simulink model "signal_tranmission"  (R2024b)
settings: Solver=ode45  StartTime=0.0  StopTime=10  FixedStep=0.000125  RelTol=1e-3
libraries: dspfdesign x500, commchan3 x1
(part 1 of 7)
settings Model: Creator=hp  LastModifiedBy=BHISMODEV

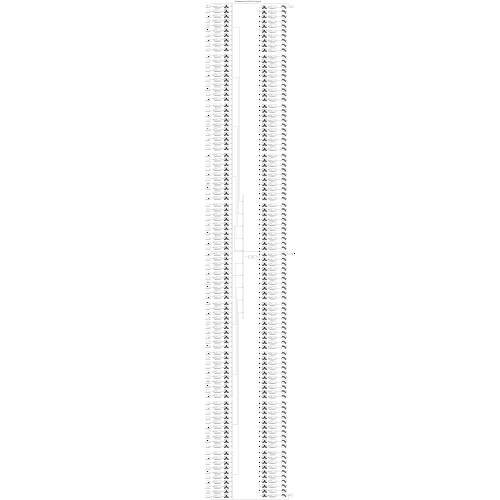
[thumbnail: Simulink's stored preview of the top-level diagram]
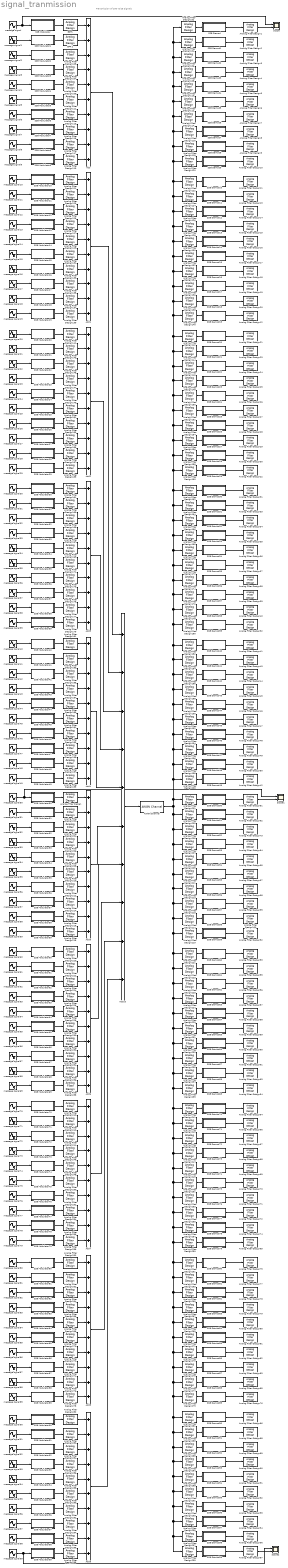
== system signal_tranmission ==
  note: Transmission of 100 Voice Signals
  AWGN Channel : commchan3/AWGN Channel  LegacyMode=off  NoiseMethod="Signal to noise ratio  (SNR)"  noiseMode="Signal to noise ratio  (SNR)"  EbNo=10  EsNo=10  SNR=80  BitsPerSymbol=1  SignalPower=1  SamplesPerSymbol=1  SymbolPeriod=1  VarianceSource=Parameter  Variance=1  RandomStream=Global stream  Seed=67  SimulateUsing=Interpreted execution
  Add{,1..10} (11 alike) : Sum  Inputs=10
  Analog Filter Design : dspfdesign/Analog Filter Design  method=Butterworth  filttype=Bandpass  N=4  Wlo=298*2*pi  Whi=302*2*pi  Rp=2  Rs=40
  Analog Filter Design{1..100} (100 alike) : dspfdesign/Analog Filter Design  method=Butterworth  filttype=Lowpass  N=4  Wlo=5*2*pi  Whi=102*2*pi  Rp=2  Rs=40
  Analog Filter Design102 : dspfdesign/Analog Filter Design  method=Butterworth  filttype=Bandpass  N=4  Wlo=98*2*pi  Whi=102*2*pi  Rp=2  Rs=40
  Analog Filter Design104 : dspfdesign/Analog Filter Design  method=Butterworth  filttype=Bandpass  N=4  Wlo=102*2*pi  Whi=106*2*pi  Rp=2  Rs=40
  Analog Filter Design105 : dspfdesign/Analog Filter Design  method=Butterworth  filttype=Bandpass  N=4  Wlo=106*2*pi  Whi=110*2*pi  Rp=2  Rs=40
  Analog Filter Design106 : dspfdesign/Analog Filter Design  method=Butterworth  filttype=Bandpass  N=4  Wlo=106*2*pi  Whi=110*2*pi  Rp=2  Rs=40
  Analog Filter Design107 : dspfdesign/Analog Filter Design  method=Butterworth  filttype=Bandpass  N=4  Wlo=110*2*pi  Whi=114*2*pi  Rp=2  Rs=40
  Analog Filter Design108 : dspfdesign/Analog Filter Design  method=Butterworth  filttype=Bandpass  N=4  Wlo=110*2*pi  Whi=114*2*pi  Rp=2  Rs=40
  Analog Filter Design109 : dspfdesign/Analog Filter Design  method=Butterworth  filttype=Bandpass  N=4  Wlo=114*2*pi  Whi=118*2*pi  Rp=2  Rs=40
  Analog Filter Design110 : dspfdesign/Analog Filter Design  method=Butterworth  filttype=Bandpass  N=4  Wlo=114*2*pi  Whi=118*2*pi  Rp=2  Rs=40
  Analog Filter Design111 : dspfdesign/Analog Filter Design  method=Butterworth  filttype=Bandpass  N=4  Wlo=118*2*pi  Whi=122*2*pi  Rp=2  Rs=40
  Analog Filter Design112 : dspfdesign/Analog Filter Design  method=Butterworth  filttype=Bandpass  N=4  Wlo=118*2*pi  Whi=122*2*pi  Rp=2  Rs=40
  Analog Filter Design113 : dspfdesign/Analog Filter Design  method=Butterworth  filttype=Bandpass  N=4  Wlo=122*2*pi  Whi=126*2*pi  Rp=2  Rs=40
  Analog Filter Design114 : dspfdesign/Analog Filter Design  method=Butterworth  filttype=Bandpass  N=4  Wlo=122*2*pi  Whi=126*2*pi  Rp=2  Rs=40
  Analog Filter Design115 : dspfdesign/Analog Filter Design  method=Butterworth  filttype=Bandpass  N=4  Wlo=126*2*pi  Whi=130*2*pi  Rp=2  Rs=40
  Analog Filter Design116 : dspfdesign/Analog Filter Design  method=Butterworth  filttype=Bandpass  N=4  Wlo=126*2*pi  Whi=130*2*pi  Rp=2  Rs=40
  Analog Filter Design117 : dspfdesign/Analog Filter Design  method=Butterworth  filttype=Bandpass  N=4  Wlo=130*2*pi  Whi=134*2*pi  Rp=2  Rs=40
  Analog Filter Design118 : dspfdesign/Analog Filter Design  method=Butterworth  filttype=Bandpass  N=4  Wlo=130*2*pi  Whi=134*2*pi  Rp=2  Rs=40
  Analog Filter Design119 : dspfdesign/Analog Filter Design  method=Butterworth  filttype=Bandpass  N=4  Wlo=134*2*pi  Whi=138*2*pi  Rp=2  Rs=40
  Analog Filter Design120 : dspfdesign/Analog Filter Design  method=Butterworth  filttype=Bandpass  N=4  Wlo=134*2*pi  Whi=138*2*pi  Rp=2  Rs=40
  Analog Filter Design121 : dspfdesign/Analog Filter Design  method=Butterworth  filttype=Bandpass  N=4  Wlo=138*2*pi  Whi=142*2*pi  Rp=2  Rs=40
  Analog Filter Design122 : dspfdesign/Analog Filter Design  method=Butterworth  filttype=Bandpass  N=4  Wlo=138*2*pi  Whi=142*2*pi  Rp=2  Rs=40
  Analog Filter Design123 : dspfdesign/Analog Filter Design  method=Butterworth  filttype=Bandpass  N=4  Wlo=142*2*pi  Whi=146*2*pi  Rp=2  Rs=40
  Analog Filter Design124 : dspfdesign/Analog Filter Design  method=Butterworth  filttype=Bandpass  N=4  Wlo=142*2*pi  Whi=146*2*pi  Rp=2  Rs=40
  Analog Filter Design125 : dspfdesign/Analog Filter Design  method=Butterworth  filttype=Bandpass  N=4  Wlo=146*2*pi  Whi=150*2*pi  Rp=2  Rs=40
  Analog Filter Design126 : dspfdesign/Analog Filter Design  method=Butterworth  filttype=Bandpass  N=4  Wlo=146*2*pi  Whi=150*2*pi  Rp=2  Rs=40
  Analog Filter Design127 : dspfdesign/Analog Filter Design  method=Butterworth  filttype=Bandpass  N=4  Wlo=150*2*pi  Whi=154*2*pi  Rp=2  Rs=40
  Analog Filter Design128 : dspfdesign/Analog Filter Design  method=Butterworth  filttype=Bandpass  N=4  Wlo=150*2*pi  Whi=154*2*pi  Rp=2  Rs=40
  Analog Filter Design129 : dspfdesign/Analog Filter Design  method=Butterworth  filttype=Bandpass  N=4  Wlo=154*2*pi  Whi=158*2*pi  Rp=2  Rs=40
  Analog Filter Design130 : dspfdesign/Analog Filter Design  method=Butterworth  filttype=Bandpass  N=4  Wlo=154*2*pi  Whi=158*2*pi  Rp=2  Rs=40
  Analog Filter Design131 : dspfdesign/Analog Filter Design  method=Butterworth  filttype=Bandpass  N=4  Wlo=158*2*pi  Whi=162*2*pi  Rp=2  Rs=40
  Analog Filter Design132 : dspfdesign/Analog Filter Design  method=Butterworth  filttype=Bandpass  N=4  Wlo=158*2*pi  Whi=162*2*pi  Rp=2  Rs=40
  Analog Filter Design133 : dspfdesign/Analog Filter Design  method=Butterworth  filttype=Bandpass  N=4  Wlo=162*2*pi  Whi=166*2*pi  Rp=2  Rs=40
  Analog Filter Design134 : dspfdesign/Analog Filter Design  method=Butterworth  filttype=Bandpass  N=4  Wlo=162*2*pi  Whi=166*2*pi  Rp=2  Rs=40
  Analog Filter Design135 : dspfdesign/Analog Filter Design  method=Butterworth  filttype=Bandpass  N=4  Wlo=166*2*pi  Whi=170*2*pi  Rp=2  Rs=40
  Analog Filter Design136 : dspfdesign/Analog Filter Design  method=Butterworth  filttype=Bandpass  N=4  Wlo=166*2*pi  Whi=170*2*pi  Rp=2  Rs=40
  Analog Filter Design137 : dspfdesign/Analog Filter Design  method=Butterworth  filttype=Bandpass  N=4  Wlo=170*2*pi  Whi=174*2*pi  Rp=2  Rs=40
  Analog Filter Design138 : dspfdesign/Analog Filter Design  method=Butterworth  filttype=Bandpass  N=4  Wlo=170*2*pi  Whi=174*2*pi  Rp=2  Rs=40
  Analog Filter Design139 : dspfdesign/Analog Filter Design  method=Butterworth  filttype=Bandpass  N=4  Wlo=174*2*pi  Whi=178*2*pi  Rp=2  Rs=40
  Analog Filter Design140 : dspfdesign/Analog Filter Design  method=Butterworth  filttype=Bandpass  N=4  Wlo=174*2*pi  Whi=178*2*pi  Rp=2  Rs=40
  Analog Filter Design141 : dspfdesign/Analog Filter Design  method=Butterworth  filttype=Bandpass  N=4  Wlo=178*2*pi  Whi=182*2*pi  Rp=2  Rs=40
  Analog Filter Design142 : dspfdesign/Analog Filter Design  method=Butterworth  filttype=Bandpass  N=4  Wlo=178*2*pi  Whi=182*2*pi  Rp=2  Rs=40
  Analog Filter Design143 : dspfdesign/Analog Filter Design  method=Butterworth  filttype=Bandpass  N=4  Wlo=182*2*pi  Whi=186*2*pi  Rp=2  Rs=40
  Analog Filter Design144 : dspfdesign/Analog Filter Design  method=Butterworth  filttype=Bandpass  N=4  Wlo=182*2*pi  Whi=186*2*pi  Rp=2  Rs=40
  Analog Filter Design145 : dspfdesign/Analog Filter Design  method=Butterworth  filttype=Bandpass  N=4  Wlo=186*2*pi  Whi=190*2*pi  Rp=2  Rs=40
  Analog Filter Design146 : dspfdesign/Analog Filter Design  method=Butterworth  filttype=Bandpass  N=4  Wlo=186*2*pi  Whi=190*2*pi  Rp=2  Rs=40
  Analog Filter Design147 : dspfdesign/Analog Filter Design  method=Butterworth  filttype=Bandpass  N=4  Wlo=190*2*pi  Whi=194*2*pi  Rp=2  Rs=40
  Analog Filter Design148 : dspfdesign/Analog Filter Design  method=Butterworth  filttype=Bandpass  N=4  Wlo=190*2*pi  Whi=194*2*pi  Rp=2  Rs=40
  Analog Filter Design149 : dspfdesign/Analog Filter Design  method=Butterworth  filttype=Bandpass  N=4  Wlo=194*2*pi  Whi=198*2*pi  Rp=2  Rs=40
  Analog Filter Design150 : dspfdesign/Analog Filter Design  method=Butterworth  filttype=Bandpass  N=4  Wlo=194*2*pi  Whi=198*2*pi  Rp=2  Rs=40
  Analog Filter Design151 : dspfdesign/Analog Filter Design  method=Butterworth  filttype=Bandpass  N=4  Wlo=198*2*pi  Whi=202*2*pi  Rp=2  Rs=40
  Analog Filter Design152 : dspfdesign/Analog Filter Design  method=Butterworth  filttype=Bandpass  N=4  Wlo=198*2*pi  Whi=202*2*pi  Rp=2  Rs=40
  Analog Filter Design153 : dspfdesign/Analog Filter Design  method=Butterworth  filttype=Bandpass  N=4  Wlo=202*2*pi  Whi=206*2*pi  Rp=2  Rs=40
  Analog Filter Design154 : dspfdesign/Analog Filter Design  method=Butterworth  filttype=Bandpass  N=4  Wlo=202*2*pi  Whi=206*2*pi  Rp=2  Rs=40
  Analog Filter Design155 : dspfdesign/Analog Filter Design  method=Butterworth  filttype=Bandpass  N=4  Wlo=206*2*pi  Whi=210*2*pi  Rp=2  Rs=40
  Analog Filter Design156 : dspfdesign/Analog Filter Design  method=Butterworth  filttype=Bandpass  N=4  Wlo=206*2*pi  Whi=210*2*pi  Rp=2  Rs=40
  Analog Filter Design157 : dspfdesign/Analog Filter Design  method=Butterworth  filttype=Bandpass  N=4  Wlo=210*2*pi  Whi=214*2*pi  Rp=2  Rs=40
  Analog Filter Design158 : dspfdesign/Analog Filter Design  method=Butterworth  filttype=Bandpass  N=4  Wlo=210*2*pi  Whi=214*2*pi  Rp=2  Rs=40
  Analog Filter Design159 : dspfdesign/Analog Filter Design  method=Butterworth  filttype=Bandpass  N=4  Wlo=214*2*pi  Whi=218*2*pi  Rp=2  Rs=40
  Analog Filter Design160 : dspfdesign/Analog Filter Design  method=Butterworth  filttype=Bandpass  N=4  Wlo=214*2*pi  Whi=218*2*pi  Rp=2  Rs=40
  Analog Filter Design161 : dspfdesign/Analog Filter Design  method=Butterworth  filttype=Bandpass  N=4  Wlo=218*2*pi  Whi=222*2*pi  Rp=2  Rs=40
  Analog Filter Design162 : dspfdesign/Analog Filter Design  method=Butterworth  filttype=Bandpass  N=4  Wlo=218*2*pi  Whi=222*2*pi  Rp=2  Rs=40
  Analog Filter Design163 : dspfdesign/Analog Filter Design  method=Butterworth  filttype=Bandpass  N=4  Wlo=222*2*pi  Whi=226*2*pi  Rp=2  Rs=40
  Analog Filter Design164 : dspfdesign/Analog Filter Design  method=Butterworth  filttype=Bandpass  N=4  Wlo=222*2*pi  Whi=226*2*pi  Rp=2  Rs=40
  Analog Filter Design165 : dspfdesign/Analog Filter Design  method=Butterworth  filttype=Bandpass  N=4  Wlo=226*2*pi  Whi=230*2*pi  Rp=2  Rs=40
  Analog Filter Design166 : dspfdesign/Analog Filter Design  method=Butterworth  filttype=Bandpass  N=4  Wlo=226*2*pi  Whi=230*2*pi  Rp=2  Rs=40
  Analog Filter Design167 : dspfdesign/Analog Filter Design  method=Butterworth  filttype=Bandpass  N=4  Wlo=230*2*pi  Whi=234*2*pi  Rp=2  Rs=40
  Analog Filter Design168 : dspfdesign/Analog Filter Design  method=Butterworth  filttype=Bandpass  N=4  Wlo=230*2*pi  Whi=234*2*pi  Rp=2  Rs=40
  Analog Filter Design169 : dspfdesign/Analog Filter Design  method=Butterworth  filttype=Bandpass  N=4  Wlo=234*2*pi  Whi=238*2*pi  Rp=2  Rs=40
  Analog Filter Design170 : dspfdesign/Analog Filter Design  method=Butterworth  filttype=Bandpass  N=4  Wlo=234*2*pi  Whi=238*2*pi  Rp=2  Rs=40
  Analog Filter Design171 : dspfdesign/Analog Filter Design  method=Butterworth  filttype=Bandpass  N=4  Wlo=238*2*pi  Whi=242*2*pi  Rp=2  Rs=40
  Analog Filter Design172 : dspfdesign/Analog Filter Design  method=Butterworth  filttype=Bandpass  N=4  Wlo=238*2*pi  Whi=242*2*pi  Rp=2  Rs=40
  Analog Filter Design173 : dspfdesign/Analog Filter Design  method=Butterworth  filttype=Bandpass  N=4  Wlo=242*2*pi  Whi=246*2*pi  Rp=2  Rs=40
  Analog Filter Design174 : dspfdesign/Analog Filter Design  method=Butterworth  filttype=Bandpass  N=4  Wlo=242*2*pi  Whi=246*2*pi  Rp=2  Rs=40
  Analog Filter Design175 : dspfdesign/Analog Filter Design  method=Butterworth  filttype=Bandpass  N=4  Wlo=246*2*pi  Whi=250*2*pi  Rp=2  Rs=40
  Analog Filter Design176 : dspfdesign/Analog Filter Design  method=Butterworth  filttype=Bandpass  N=4  Wlo=246*2*pi  Whi=250*2*pi  Rp=2  Rs=40
  Analog Filter Design177 : dspfdesign/Analog Filter Design  method=Butterworth  filttype=Bandpass  N=4  Wlo=250*2*pi  Whi=254*2*pi  Rp=2  Rs=40
  Analog Filter Design178 : dspfdesign/Analog Filter Design  method=Butterworth  filttype=Bandpass  N=4  Wlo=250*2*pi  Whi=254*2*pi  Rp=2  Rs=40
  Analog Filter Design179 : dspfdesign/Analog Filter Design  method=Butterworth  filttype=Bandpass  N=4  Wlo=254*2*pi  Whi=258*2*pi  Rp=2  Rs=40
  Analog Filter Design180 : dspfdesign/Analog Filter Design  method=Butterworth  filttype=Bandpass  N=4  Wlo=254*2*pi  Whi=258*2*pi  Rp=2  Rs=40
  Analog Filter Design181 : dspfdesign/Analog Filter Design  method=Butterworth  filttype=Bandpass  N=4  Wlo=258*2*pi  Whi=262*2*pi  Rp=2  Rs=40
  Analog Filter Design182 : dspfdesign/Analog Filter Design  method=Butterworth  filttype=Bandpass  N=4  Wlo=258*2*pi  Whi=262*2*pi  Rp=2  Rs=40
  Analog Filter Design183 : dspfdesign/Analog Filter Design  method=Butterworth  filttype=Bandpass  N=4  Wlo=262*2*pi  Whi=266*2*pi  Rp=2  Rs=40
  Analog Filter Design184 : dspfdesign/Analog Filter Design  method=Butterworth  filttype=Bandpass  N=4  Wlo=262*2*pi  Whi=266*2*pi  Rp=2  Rs=40
  Analog Filter Design185 : dspfdesign/Analog Filter Design  method=Butterworth  filttype=Bandpass  N=4  Wlo=266*2*pi  Whi=270*2*pi  Rp=2  Rs=40
  Analog Filter Design186 : dspfdesign/Analog Filter Design  method=Butterworth  filttype=Bandpass  N=4  Wlo=266*2*pi  Whi=270*2*pi  Rp=2  Rs=40
  Analog Filter Design187 : dspfdesign/Analog Filter Design  method=Butterworth  filttype=Bandpass  N=4  Wlo=270*2*pi  Whi=274*2*pi  Rp=2  Rs=40
  Analog Filter Design188 : dspfdesign/Analog Filter Design  method=Butterworth  filttype=Bandpass  N=4  Wlo=270*2*pi  Whi=274*2*pi  Rp=2  Rs=40
  Analog Filter Design189 : dspfdesign/Analog Filter Design  method=Butterworth  filttype=Bandpass  N=4  Wlo=274*2*pi  Whi=278*2*pi  Rp=2  Rs=40
  Analog Filter Design190 : dspfdesign/Analog Filter Design  method=Butterworth  filttype=Bandpass  N=4  Wlo=274*2*pi  Whi=278*2*pi  Rp=2  Rs=40
  Analog Filter Design191 : dspfdesign/Analog Filter Design  method=Butterworth  filttype=Bandpass  N=4  Wlo=278*2*pi  Whi=282*2*pi  Rp=2  Rs=40
  Analog Filter Design192 : dspfdesign/Analog Filter Design  method=Butterworth  filttype=Bandpass  N=4  Wlo=278*2*pi  Whi=282*2*pi  Rp=2  Rs=40
  Analog Filter Design193 : dspfdesign/Analog Filter Design  method=Butterworth  filttype=Bandpass  N=4  Wlo=282*2*pi  Whi=286*2*pi  Rp=2  Rs=40
  Analog Filter Design194 : dspfdesign/Analog Filter Design  method=Butterworth  filttype=Bandpass  N=4  Wlo=282*2*pi  Whi=286*2*pi  Rp=2  Rs=40
  Analog Filter Design195 : dspfdesign/Analog Filter Design  method=Butterworth  filttype=Bandpass  N=4  Wlo=286*2*pi  Whi=290*2*pi  Rp=2  Rs=40
  Analog Filter Design196 : dspfdesign/Analog Filter Design  method=Butterworth  filttype=Bandpass  N=4  Wlo=286*2*pi  Whi=290*2*pi  Rp=2  Rs=40
  Analog Filter Design197 : dspfdesign/Analog Filter Design  method=Butterworth  filttype=Bandpass  N=4  Wlo=290*2*pi  Whi=294*2*pi  Rp=2  Rs=40
  Analog Filter Design198 : dspfdesign/Analog Filter Design  method=Butterworth  filttype=Bandpass  N=4  Wlo=290*2*pi  Whi=294*2*pi  Rp=2  Rs=40
  Analog Filter Design199 : dspfdesign/Analog Filter Design  method=Butterworth  filttype=Bandpass  N=4  Wlo=294*2*pi  Whi=298*2*pi  Rp=2  Rs=40
  Analog Filter Design200 : dspfdesign/Analog Filter Design  method=Butterworth  filttype=Bandpass  N=4  Wlo=294*2*pi  Whi=298*2*pi  Rp=2  Rs=40
  Analog Filter Design201 : dspfdesign/Analog Filter Design  method=Butterworth  filttype=Bandpass  N=4  Wlo=298*2*pi  Whi=302*2*pi  Rp=2  Rs=40
  Analog Filter Design202 : dspfdesign/Analog Filter Design  method=Butterworth  filttype=Bandpass  N=4  Wlo=302*2*pi  Whi=306*2*pi  Rp=2  Rs=40
  Analog Filter Design203 : dspfdesign/Analog Filter Design  method=Butterworth  filttype=Bandpass  N=4  Wlo=302*2*pi  Whi=306*2*pi  Rp=2  Rs=40
  Analog Filter Design204 : dspfdesign/Analog Filter Design  method=Butterworth  filttype=Bandpass  N=4  Wlo=306*2*pi  Whi=310*2*pi  Rp=2  Rs=40
  Analog Filter Design205 : dspfdesign/Analog Filter Design  method=Butterworth  filttype=Bandpass  N=4  Wlo=306*2*pi  Whi=310*2*pi  Rp=2  Rs=40
  Analog Filter Design206 : dspfdesign/Analog Filter Design  method=Butterworth  filttype=Bandpass  N=4  Wlo=310*2*pi  Whi=314*2*pi  Rp=2  Rs=40
  Analog Filter Design207 : dspfdesign/Analog Filter Design  method=Butterworth  filttype=Bandpass  N=4  Wlo=310*2*pi  Whi=314*2*pi  Rp=2  Rs=40
  Analog Filter Design208 : dspfdesign/Analog Filter Design  method=Butterworth  filttype=Bandpass  N=4  Wlo=314*2*pi  Whi=318*2*pi  Rp=2  Rs=40
  Analog Filter Design209 : dspfdesign/Analog Filter Design  method=Butterworth  filttype=Bandpass  N=4  Wlo=314*2*pi  Whi=318*2*pi  Rp=2  Rs=40
  Analog Filter Design210 : dspfdesign/Analog Filter Design  method=Butterworth  filttype=Bandpass  N=4  Wlo=318*2*pi  Whi=322*2*pi  Rp=2  Rs=40
  Analog Filter Design211 : dspfdesign/Analog Filter Design  method=Butterworth  filttype=Bandpass  N=4  Wlo=318*2*pi  Whi=322*2*pi  Rp=2  Rs=40
  Analog Filter Design212 : dspfdesign/Analog Filter Design  method=Butterworth  filttype=Bandpass  N=4  Wlo=322*2*pi  Whi=326*2*pi  Rp=2  Rs=40
  Analog Filter Design213 : dspfdesign/Analog Filter Design  method=Butterworth  filttype=Bandpass  N=4  Wlo=322*2*pi  Whi=326*2*pi  Rp=2  Rs=40
  Analog Filter Design214 : dspfdesign/Analog Filter Design  method=Butterworth  filttype=Bandpass  N=4  Wlo=326*2*pi  Whi=330*2*pi  Rp=2  Rs=40
  Analog Filter Design215 : dspfdesign/Analog Filter Design  method=Butterworth  filttype=Bandpass  N=4  Wlo=326*2*pi  Whi=330*2*pi  Rp=2  Rs=40
  Analog Filter Design216 : dspfdesign/Analog Filter Design  method=Butterworth  filttype=Bandpass  N=4  Wlo=330*2*pi  Whi=334*2*pi  Rp=2  Rs=40
  Analog Filter Design217 : dspfdesign/Analog Filter Design  method=Butterworth  filttype=Bandpass  N=4  Wlo=330*2*pi  Whi=334*2*pi  Rp=2  Rs=40
  Analog Filter Design218 : dspfdesign/Analog Filter Design  method=Butterworth  filttype=Bandpass  N=4  Wlo=334*2*pi  Whi=338*2*pi  Rp=2  Rs=40
  Analog Filter Design219 : dspfdesign/Analog Filter Design  method=Butterworth  filttype=Bandpass  N=4  Wlo=334*2*pi  Whi=338*2*pi  Rp=2  Rs=40
  Analog Filter Design220 : dspfdesign/Analog Filter Design  method=Butterworth  filttype=Bandpass  N=4  Wlo=338*2*pi  Whi=342*2*pi  Rp=2  Rs=40
  Analog Filter Design221 : dspfdesign/Analog Filter Design  method=Butterworth  filttype=Bandpass  N=4  Wlo=338*2*pi  Whi=342*2*pi  Rp=2  Rs=40
  Analog Filter Design222 : dspfdesign/Analog Filter Design  method=Butterworth  filttype=Bandpass  N=4  Wlo=342*2*pi  Whi=346*2*pi  Rp=2  Rs=40
  Analog Filter Design223 : dspfdesign/Analog Filter Design  method=Butterworth  filttype=Bandpass  N=4  Wlo=342*2*pi  Whi=346*2*pi  Rp=2  Rs=40
  Analog Filter Design224 : dspfdesign/Analog Filter Design  method=Butterworth  filttype=Bandpass  N=4  Wlo=346*2*pi  Whi=350*2*pi  Rp=2  Rs=40
  Analog Filter Design225 : dspfdesign/Analog Filter Design  method=Butterworth  filttype=Bandpass  N=4  Wlo=346*2*pi  Whi=350*2*pi  Rp=2  Rs=40
  Analog Filter Design226 : dspfdesign/Analog Filter Design  method=Butterworth  filttype=Bandpass  N=4  Wlo=350*2*pi  Whi=354*2*pi  Rp=2  Rs=40
  Analog Filter Design227 : dspfdesign/Analog Filter Design  method=Butterworth  filttype=Bandpass  N=4  Wlo=350*2*pi  Whi=354*2*pi  Rp=2  Rs=40
  Analog Filter Design228 : dspfdesign/Analog Filter Design  method=Butterworth  filttype=Bandpass  N=4  Wlo=354*2*pi  Whi=358*2*pi  Rp=2  Rs=40
  Analog Filter Design229 : dspfdesign/Analog Filter Design  method=Butterworth  filttype=Bandpass  N=4  Wlo=354*2*pi  Whi=358*2*pi  Rp=2  Rs=40
  Analog Filter Design230 : dspfdesign/Analog Filter Design  method=Butterworth  filttype=Bandpass  N=4  Wlo=358*2*pi  Whi=362*2*pi  Rp=2  Rs=40
  Analog Filter Design231 : dspfdesign/Analog Filter Design  method=Butterworth  filttype=Bandpass  N=4  Wlo=358*2*pi  Whi=362*2*pi  Rp=2  Rs=40
  Analog Filter Design232 : dspfdesign/Analog Filter Design  method=Butterworth  filttype=Bandpass  N=4  Wlo=362*2*pi  Whi=366*2*pi  Rp=2  Rs=40
  Analog Filter Design233 : dspfdesign/Analog Filter Design  method=Butterworth  filttype=Bandpass  N=4  Wlo=362*2*pi  Whi=366*2*pi  Rp=2  Rs=40
  Analog Filter Design234 : dspfdesign/Analog Filter Design  method=Butterworth  filttype=Bandpass  N=4  Wlo=366*2*pi  Whi=370*2*pi  Rp=2  Rs=40
  Analog Filter Design235 : dspfdesign/Analog Filter Design  method=Butterworth  filttype=Bandpass  N=4  Wlo=366*2*pi  Whi=370*2*pi  Rp=2  Rs=40
  Analog Filter Design236 : dspfdesign/Analog Filter Design  method=Butterworth  filttype=Bandpass  N=4  Wlo=370*2*pi  Whi=374*2*pi  Rp=2  Rs=40
  Analog Filter Design237 : dspfdesign/Analog Filter Design  method=Butterworth  filttype=Bandpass  N=4  Wlo=370*2*pi  Whi=374*2*pi  Rp=2  Rs=40
  Analog Filter Design238 : dspfdesign/Analog Filter Design  method=Butterworth  filttype=Bandpass  N=4  Wlo=374*2*pi  Whi=378*2*pi  Rp=2  Rs=40
  Analog Filter Design239 : dspfdesign/Analog Filter Design  method=Butterworth  filttype=Bandpass  N=4  Wlo=374*2*pi  Whi=378*2*pi  Rp=2  Rs=40
  Analog Filter Design240 : dspfdesign/Analog Filter Design  method=Butterworth  filttype=Bandpass  N=4  Wlo=378*2*pi  Whi=382*2*pi  Rp=2  Rs=40
  Analog Filter Design241 : dspfdesign/Analog Filter Design  method=Butterworth  filttype=Bandpass  N=4  Wlo=378*2*pi  Whi=382*2*pi  Rp=2  Rs=40
  Analog Filter Design242 : dspfdesign/Analog Filter Design  method=Butterworth  filttype=Bandpass  N=4  Wlo=382*2*pi  Whi=386*2*pi  Rp=2  Rs=40
  Analog Filter Design243 : dspfdesign/Analog Filter Design  method=Butterworth  filttype=Bandpass  N=4  Wlo=382*2*pi  Whi=386*2*pi  Rp=2  Rs=40
  Analog Filter Design244 : dspfdesign/Analog Filter Design  method=Butterworth  filttype=Bandpass  N=4  Wlo=386*2*pi  Whi=390*2*pi  Rp=2  Rs=40
  Analog Filter Design245 : dspfdesign/Analog Filter Design  method=Butterworth  filttype=Bandpass  N=4  Wlo=386*2*pi  Whi=390*2*pi  Rp=2  Rs=40
  Analog Filter Design246 : dspfdesign/Analog Filter Design  method=Butterworth  filttype=Bandpass  N=4  Wlo=390*2*pi  Whi=394*2*pi  Rp=2  Rs=40
  Analog Filter Design247 : dspfdesign/Analog Filter Design  method=Butterworth  filttype=Bandpass  N=4  Wlo=390*2*pi  Whi=394*2*pi  Rp=2  Rs=40
  Analog Filter Design248 : dspfdesign/Analog Filter Design  method=Butterworth  filttype=Bandpass  N=4  Wlo=394*2*pi  Whi=398*2*pi  Rp=2  Rs=40
  Analog Filter Design249 : dspfdesign/Analog Filter Design  method=Butterworth  filttype=Bandpass  N=4  Wlo=394*2*pi  Whi=398*2*pi  Rp=2  Rs=40
  Analog Filter Design250 : dspfdesign/Analog Filter Design  method=Butterworth  filttype=Bandpass  N=4  Wlo=398*2*pi  Whi=402*2*pi  Rp=2  Rs=40
  Analog Filter Design251 : dspfdesign/Analog Filter Design  method=Butterworth  filttype=Bandpass  N=4  Wlo=398*2*pi  Whi=402*2*pi  Rp=2  Rs=40
  Analog Filter Design252 : dspfdesign/Analog Filter Design  method=Butterworth  filttype=Bandpass  N=4  Wlo=402*2*pi  Whi=406*2*pi  Rp=2  Rs=40
  Analog Filter Design253 : dspfdesign/Analog Filter Design  method=Butterworth  filttype=Bandpass  N=4  Wlo=402*2*pi  Whi=406*2*pi  Rp=2  Rs=40
  Analog Filter Design254 : dspfdesign/Analog Filter Design  method=Butterworth  filttype=Bandpass  N=4  Wlo=406*2*pi  Whi=410*2*pi  Rp=2  Rs=40
  Analog Filter Design255 : dspfdesign/Analog Filter Design  method=Butterworth  filttype=Bandpass  N=4  Wlo=406*2*pi  Whi=410*2*pi  Rp=2  Rs=40
  Analog Filter Design256 : dspfdesign/Analog Filter Design  method=Butterworth  filttype=Bandpass  N=4  Wlo=410*2*pi  Whi=414*2*pi  Rp=2  Rs=40
  Analog Filter Design257 : dspfdesign/Analog Filter Design  method=Butterworth  filttype=Bandpass  N=4  Wlo=410*2*pi  Whi=414*2*pi  Rp=2  Rs=40
  Analog Filter Design258 : dspfdesign/Analog Filter Design  method=Butterworth  filttype=Bandpass  N=4  Wlo=414*2*pi  Whi=418*2*pi  Rp=2  Rs=40
  Analog Filter Design259 : dspfdesign/Analog Filter Design  method=Butterworth  filttype=Bandpass  N=4  Wlo=414*2*pi  Whi=418*2*pi  Rp=2  Rs=40
  Analog Filter Design260 : dspfdesign/Analog Filter Design  method=Butterworth  filttype=Bandpass  N=4  Wlo=418*2*pi  Whi=422*2*pi  Rp=2  Rs=40
  Analog Filter Design261 : dspfdesign/Analog Filter Design  method=Butterworth  filttype=Bandpass  N=4  Wlo=418*2*pi  Whi=422*2*pi  Rp=2  Rs=40
  Analog Filter Design262 : dspfdesign/Analog Filter Design  method=Butterworth  filttype=Bandpass  N=4  Wlo=422*2*pi  Whi=426*2*pi  Rp=2  Rs=40
  Analog Filter Design263 : dspfdesign/Analog Filter Design  method=Butterworth  filttype=Bandpass  N=4  Wlo=422*2*pi  Whi=426*2*pi  Rp=2  Rs=40
  Analog Filter Design264 : dspfdesign/Analog Filter Design  method=Butterworth  filttype=Bandpass  N=4  Wlo=426*2*pi  Whi=430*2*pi  Rp=2  Rs=40
  Analog Filter Design265 : dspfdesign/Analog Filter Design  method=Butterworth  filttype=Bandpass  N=4  Wlo=426*2*pi  Whi=430*2*pi  Rp=2  Rs=40
  Analog Filter Design266 : dspfdesign/Analog Filter Design  method=Butterworth  filttype=Bandpass  N=4  Wlo=430*2*pi  Whi=434*2*pi  Rp=2  Rs=40
  Analog Filter Design267 : dspfdesign/Analog Filter Design  method=Butterworth  filttype=Bandpass  N=4  Wlo=430*2*pi  Whi=434*2*pi  Rp=2  Rs=40
  Analog Filter Design268 : dspfdesign/Analog Filter Design  method=Butterworth  filttype=Bandpass  N=4  Wlo=434*2*pi  Whi=438*2*pi  Rp=2  Rs=40
  Analog Filter Design269 : dspfdesign/Analog Filter Design  method=Butterworth  filttype=Bandpass  N=4  Wlo=434*2*pi  Whi=438*2*pi  Rp=2  Rs=40
  Analog Filter Design270 : dspfdesign/Analog Filter Design  method=Butterworth  filttype=Bandpass  N=4  Wlo=438*2*pi  Whi=442*2*pi  Rp=2  Rs=40
  Analog Filter Design271 : dspfdesign/Analog Filter Design  method=Butterworth  filttype=Bandpass  N=4  Wlo=438*2*pi  Whi=442*2*pi  Rp=2  Rs=40
  Analog Filter Design272 : dspfdesign/Analog Filter Design  method=Butterworth  filttype=Bandpass  N=4  Wlo=442*2*pi  Whi=446*2*pi  Rp=2  Rs=40
  Analog Filter Design273 : dspfdesign/Analog Filter Design  method=Butterworth  filttype=Bandpass  N=4  Wlo=442*2*pi  Whi=446*2*pi  Rp=2  Rs=40
  Analog Filter Design274 : dspfdesign/Analog Filter Design  method=Butterworth  filttype=Bandpass  N=4  Wlo=446*2*pi  Whi=450*2*pi  Rp=2  Rs=40
  Analog Filter Design275 : dspfdesign/Analog Filter Design  method=Butterworth  filttype=Bandpass  N=4  Wlo=446*2*pi  Whi=450*2*pi  Rp=2  Rs=40
  Analog Filter Design276 : dspfdesign/Analog Filter Design  method=Butterworth  filttype=Bandpass  N=4  Wlo=450*2*pi  Whi=454*2*pi  Rp=2  Rs=40
  Analog Filter Design277 : dspfdesign/Analog Filter Design  method=Butterworth  filttype=Bandpass  N=4  Wlo=450*2*pi  Whi=454*2*pi  Rp=2  Rs=40
  Analog Filter Design278 : dspfdesign/Analog Filter Design  method=Butterworth  filttype=Bandpass  N=4  Wlo=454*2*pi  Whi=458*2*pi  Rp=2  Rs=40
  Analog Filter Design279 : dspfdesign/Analog Filter Design  method=Butterworth  filttype=Bandpass  N=4  Wlo=454*2*pi  Whi=458*2*pi  Rp=2  Rs=40
  Analog Filter Design280 : dspfdesign/Analog Filter Design  method=Butterworth  filttype=Bandpass  N=4  Wlo=458*2*pi  Whi=462*2*pi  Rp=2  Rs=40
  Analog Filter Design281 : dspfdesign/Analog Filter Design  method=Butterworth  filttype=Bandpass  N=4  Wlo=458*2*pi  Whi=462*2*pi  Rp=2  Rs=40
  Analog Filter Design282 : dspfdesign/Analog Filter Design  method=Butterworth  filttype=Bandpass  N=4  Wlo=462*2*pi  Whi=466*2*pi  Rp=2  Rs=40
  Analog Filter Design283 : dspfdesign/Analog Filter Design  method=Butterworth  filttype=Bandpass  N=4  Wlo=462*2*pi  Whi=466*2*pi  Rp=2  Rs=40
  Analog Filter Design284 : dspfdesign/Analog Filter Design  method=Butterworth  filttype=Bandpass  N=4  Wlo=466*2*pi  Whi=470*2*pi  Rp=2  Rs=40
  Analog Filter Design285 : dspfdesign/Analog Filter Design  method=Butterworth  filttype=Bandpass  N=4  Wlo=466*2*pi  Whi=470*2*pi  Rp=2  Rs=40
  Analog Filter Design286 : dspfdesign/Analog Filter Design  method=Butterworth  filttype=Bandpass  N=4  Wlo=470*2*pi  Whi=474*2*pi  Rp=2  Rs=40
  Analog Filter Design287 : dspfdesign/Analog Filter Design  method=Butterworth  filttype=Bandpass  N=4  Wlo=470*2*pi  Whi=474*2*pi  Rp=2  Rs=40
  Analog Filter Design288 : dspfdesign/Analog Filter Design  method=Butterworth  filttype=Bandpass  N=4  Wlo=474*2*pi  Whi=478*2*pi  Rp=2  Rs=40
  Analog Filter Design289 : dspfdesign/Analog Filter Design  method=Butterworth  filttype=Bandpass  N=4  Wlo=474*2*pi  Whi=478*2*pi  Rp=2  Rs=40
  Analog Filter Design290 : dspfdesign/Analog Filter Design  method=Butterworth  filttype=Bandpass  N=4  Wlo=478*2*pi  Whi=482*2*pi  Rp=2  Rs=40
  Analog Filter Design291 : dspfdesign/Analog Filter Design  method=Butterworth  filttype=Bandpass  N=4  Wlo=478*2*pi  Whi=482*2*pi  Rp=2  Rs=40
  Analog Filter Design292 : dspfdesign/Analog Filter Design  method=Butterworth  filttype=Bandpass  N=4  Wlo=482*2*pi  Whi=486*2*pi  Rp=2  Rs=40
  Analog Filter Design293 : dspfdesign/Analog Filter Design  method=Butterworth  filttype=Bandpass  N=4  Wlo=482*2*pi  Whi=486*2*pi  Rp=2  Rs=40
  Analog Filter Design294 : dspfdesign/Analog Filter Design  method=Butterworth  filttype=Bandpass  N=4  Wlo=486*2*pi  Whi=490*2*pi  Rp=2  Rs=40
  Analog Filter Design295 : dspfdesign/Analog Filter Design  method=Butterworth  filttype=Bandpass  N=4  Wlo=486*2*pi  Whi=490*2*pi  Rp=2  Rs=40
  Analog Filter Design296 : dspfdesign/Analog Filter Design  method=Butterworth  filttype=Bandpass  N=4  Wlo=490*2*pi  Whi=494*2*pi  Rp=2  Rs=40
  Analog Filter Design297 : dspfdesign/Analog Filter Design  method=Butterworth  filttype=Bandpass  N=4  Wlo=490*2*pi  Whi=494*2*pi  Rp=2  Rs=40
  Analog Filter Design298 : dspfdesign/Analog Filter Design  method=Butterworth  filttype=Bandpass  N=4  Wlo=494*2*pi  Whi=498*2*pi  Rp=2  Rs=40
  Analog Filter Design299 : dspfdesign/Analog Filter Design  method=Butterworth  filttype=Bandpass  N=4  Wlo=494*2*pi  Whi=498*2*pi  Rp=2  Rs=40
  BPF 2 : dspfdesign/Analog Filter Design  method=Butterworth  filttype=Bandpass  N=4  Wlo=102*2*pi  Whi=106*2*pi  Rp=2  Rs=40
  BPF1 : dspfdesign/Analog Filter Design  method=Butterworth  filttype=Bandpass  N=4  Wlo=98*2*pi  Whi=102*2*pi  Rp=2  Rs=40
  SSB Demod : Subsystem
  SSB Demod1 : Subsystem
  SSB Demod10 : Subsystem
  SSB Demod11 : Subsystem
  SSB Demod12 : Subsystem
  SSB Demod13 : Subsystem
  SSB Demod14 : Subsystem
  SSB Demod15 : Subsystem
  SSB Demod16 : Subsystem
  SSB Demod17 : Subsystem
  SSB Demod18 : Subsystem
  SSB Demod19 : Subsystem
  SSB Demod2 : Subsystem
  SSB Demod20 : Subsystem
  SSB Demod21 : Subsystem
  SSB Demod22 : Subsystem
  SSB Demod23 : Subsystem
  SSB Demod24 : Subsystem
  SSB Demod25 : Subsystem
  SSB Demod26 : Subsystem
  SSB Demod27 : Subsystem
  SSB Demod28 : Subsystem
  SSB Demod29 : Subsystem
  SSB Demod3 : Subsystem
  SSB Demod30 : Subsystem
  SSB Demod31 : Subsystem
  SSB Demod32 : Subsystem
  SSB Demod33 : Subsystem
  SSB Demod34 : Subsystem
  SSB Demod35 : Subsystem
  SSB Demod36 : Subsystem
  SSB Demod37 : Subsystem
  SSB Demod38 : Subsystem
  SSB Demod39 : Subsystem
  SSB Demod4 : Subsystem
  SSB Demod40 : Subsystem
  SSB Demod41 : Subsystem
  SSB Demod42 : Subsystem
  SSB Demod43 : Subsystem
  SSB Demod44 : Subsystem
  SSB Demod45 : Subsystem
  SSB Demod46 : Subsystem
  SSB Demod47 : Subsystem
  SSB Demod48 : Subsystem
  SSB Demod49 : Subsystem
  SSB Demod5 : Subsystem
  SSB Demod50 : Subsystem
  SSB Demod51 : Subsystem
  SSB Demod52 : Subsystem
  SSB Demod53 : Subsystem
  SSB Demod54 : Subsystem
  SSB Demod55 : Subsystem
  SSB Demod56 : Subsystem
  SSB Demod57 : Subsystem
  SSB Demod58 : Subsystem
  SSB Demod59 : Subsystem
  SSB Demod6 : Subsystem
  SSB Demod60 : Subsystem
  SSB Demod61 : Subsystem
  SSB Demod62 : Subsystem
  SSB Demod63 : Subsystem
  SSB Demod64 : Subsystem
  SSB Demod65 : Subsystem
  SSB Demod66 : Subsystem
  SSB Demod67 : Subsystem
  SSB Demod68 : Subsystem
  SSB Demod69 : Subsystem
  SSB Demod7 : Subsystem
  SSB Demod70 : Subsystem
  SSB Demod71 : Subsystem
  SSB Demod72 : Subsystem
  SSB Demod73 : Subsystem
  SSB Demod74 : Subsystem
  SSB Demod75 : Subsystem
  SSB Demod76 : Subsystem
  SSB Demod77 : Subsystem
  SSB Demod78 : Subsystem
  SSB Demod79 : Subsystem
  SSB Demod8 : Subsystem
  SSB Demod80 : Subsystem
  SSB Demod81 : Subsystem
  SSB Demod82 : Subsystem
  SSB Demod83 : Subsystem
  SSB Demod84 : Subsystem
  SSB Demod85 : Subsystem
  SSB Demod86 : Subsystem
  SSB Demod87 : Subsystem
  SSB Demod88 : Subsystem
  SSB Demod89 : Subsystem
  SSB Demod9 : Subsystem
  SSB Demod90 : Subsystem
  SSB Demod91 : Subsystem
  SSB Demod92 : Subsystem
  SSB Demod93 : Subsystem
  SSB Demod94 : Subsystem
  SSB Demod95 : Subsystem
  SSB Demod96 : Subsystem
  SSB Demod97 : Subsystem
  SSB Demod98 : Subsystem
  SSB Demod99 : Subsystem
  SSB Modulator : Subsystem
  SSB Modulator1 : Subsystem
  SSB Modulator10 : Subsystem
  SSB Modulator11 : Subsystem
  SSB Modulator12 : Subsystem
  SSB Modulator13 : Subsystem
  SSB Modulator14 : Subsystem
  SSB Modulator15 : Subsystem
  SSB Modulator16 : Subsystem
  SSB Modulator17 : Subsystem
  SSB Modulator18 : Subsystem
  SSB Modulator19 : Subsystem
  SSB Modulator2 : Subsystem
  SSB Modulator20 : Subsystem
  SSB Modulator21 : Subsystem
  SSB Modulator22 : Subsystem
  SSB Modulator23 : Subsystem
  SSB Modulator24 : Subsystem
  SSB Modulator25 : Subsystem
  SSB Modulator26 : Subsystem
  SSB Modulator27 : Subsystem
  SSB Modulator28 : Subsystem
  SSB Modulator29 : Subsystem
  SSB Modulator3 : Subsystem
  SSB Modulator30 : Subsystem
  SSB Modulator31 : Subsystem
  SSB Modulator32 : Subsystem
  SSB Modulator33 : Subsystem
  SSB Modulator34 : Subsystem
  SSB Modulator35 : Subsystem
  SSB Modulator36 : Subsystem
  SSB Modulator37 : Subsystem
  SSB Modulator38 : Subsystem
  SSB Modulator39 : Subsystem
  SSB Modulator4 : Subsystem
  SSB Modulator40 : Subsystem
  SSB Modulator41 : Subsystem
  SSB Modulator42 : Subsystem
  SSB Modulator43 : Subsystem
  SSB Modulator44 : Subsystem
  SSB Modulator45 : Subsystem
  SSB Modulator46 : Subsystem
  SSB Modulator47 : Subsystem
  SSB Modulator48 : Subsystem
  SSB Modulator49 : Subsystem
  SSB Modulator5 : Subsystem
  SSB Modulator50 : Subsystem
  SSB Modulator51 : Subsystem
  SSB Modulator52 : Subsystem
  SSB Modulator53 : Subsystem
  SSB Modulator54 : Subsystem
  SSB Modulator55 : Subsystem
  SSB Modulator56 : Subsystem
  SSB Modulator57 : Subsystem
  SSB Modulator58 : Subsystem
  SSB Modulator59 : Subsystem
  SSB Modulator6 : Subsystem
  SSB Modulator60 : Subsystem
  SSB Modulator61 : Subsystem
  SSB Modulator62 : Subsystem
  SSB Modulator63 : Subsystem
  SSB Modulator64 : Subsystem
  SSB Modulator65 : Subsystem
  SSB Modulator66 : Subsystem
  SSB Modulator67 : Subsystem
  SSB Modulator68 : Subsystem
  SSB Modulator69 : Subsystem
  SSB Modulator7 : Subsystem
  SSB Modulator70 : Subsystem
  SSB Modulator71 : Subsystem
  SSB Modulator72 : Subsystem
  SSB Modulator73 : Subsystem
  SSB Modulator74 : Subsystem
  SSB Modulator75 : Subsystem
  SSB Modulator76 : Subsystem
  SSB Modulator77 : Subsystem
  SSB Modulator78 : Subsystem
  SSB Modulator79 : Subsystem
  SSB Modulator8 : Subsystem
  SSB Modulator80 : Subsystem
  SSB Modulator81 : Subsystem
  SSB Modulator82 : Subsystem
  SSB Modulator83 : Subsystem
  SSB Modulator84 : Subsystem
  SSB Modulator85 : Subsystem
  SSB Modulator86 : Subsystem
  SSB Modulator87 : Subsystem
  SSB Modulator88 : Subsystem
  SSB Modulator89 : Subsystem
  SSB Modulator9 : Subsystem
  SSB Modulator90 : Subsystem
  SSB Modulator91 : Subsystem
  SSB Modulator92 : Subsystem
  SSB Modulator93 : Subsystem
  SSB Modulator94 : Subsystem
  SSB Modulator95 : Subsystem
  SSB Modulator96 : Subsystem
  SSB Modulator97 : Subsystem
  SSB Modulator98 : Subsystem
  SSB Modulator99 : Subsystem
  Scope : Scope  NumInputPorts=2
  Scope1 : Scope  NumInputPorts=2
  Scope2 : Scope  NumInputPorts=2
  message signal{,1..99} (100 alike) : Sin  Frequency=4*2*pi  SampleTime=0
  wires:
  Analog Filter Design216/1 -> Add5/9
  Analog Filter Design220/1 -> Add6/1
  Analog Filter Design280/1 -> Add9/1
  Analog Filter Design286/1 -> Add9/4
  Analog Filter Design287/1 -> SSB Demod93/1(Input Signal)
  Analog Filter Design148/1 -> SSB Demod23/1(Input Signal)
  Analog Filter Design147/1 -> Add2/4
  Analog Filter Design157/1 -> Add2/9
  Analog Filter Design213/1 -> SSB Demod56/1(Input Signal)
  Analog Filter Design251/1 -> SSB Demod75/1(Input Signal)
  Analog Filter Design206/1 -> Add5/4
  Analog Filter Design207/1 -> SSB Demod53/1(Input Signal)
  Analog Filter Design153/1 -> Add2/7
  Analog Filter Design146/1 -> SSB Demod22/1(Input Signal)
  Analog Filter Design142/1 -> SSB Demod20/1(Input Signal)
  Analog Filter Design255/1 -> SSB Demod77/1(Input Signal)
  Analog Filter Design170/1 -> SSB Demod34/1(Input Signal)
  Analog Filter Design289/1 -> SSB Demod94/1(Input Signal)
  Analog Filter Design138/1 -> SSB Demod18/1(Input Signal)
  Analog Filter Design248/1 -> Add7/5
  Analog Filter Design145/1 -> Add2/3
  Analog Filter Design260/1 -> Add8/1
  Analog Filter Design113/1 -> Add/7
  Analog Filter Design171/1 -> Add3/6
  Analog Filter Design109/1 -> Add/5
  Analog Filter Design107/1 -> Add/4
  Analog Filter Design266/1 -> Add8/4
  Analog Filter Design185/1 -> Add4/3
  Analog Filter Design203/1 -> SSB Demod51/1(Input Signal)
  Analog Filter Design284/1 -> Add9/3
  Analog Filter Design182/1 -> SSB Demod40/1(Input Signal)
  Analog Filter Design133/1 -> Add1/7
  Analog Filter Design130/1 -> SSB Demod14/1(Input Signal)
  Analog Filter Design224/1 -> Add6/3
  Analog Filter Design238/1 -> Add6/10
  Analog Filter Design195/1 -> Add4/8
  Analog Filter Design210/1 -> Add5/6
  Analog Filter Design232/1 -> Add6/7
  Analog Filter Design181/1 -> Add4/1
  Analog Filter Design219/1 -> SSB Demod59/1(Input Signal)
  Analog Filter Design115/1 -> Add/8
  Analog Filter Design1/1 -> Scope/2
  Analog Filter Design202/1 -> Add5/2
  Analog Filter Design172/1 -> SSB Demod35/1(Input Signal)
  Analog Filter Design180/1 -> SSB Demod39/1(Input Signal)
  Analog Filter Design51/1 -> Scope1/2
  Analog Filter Design189/1 -> Add4/5
  Analog Filter Design155/1 -> Add2/8
  Analog Filter Design183/1 -> Add4/2
  Analog Filter Design277/1 -> SSB Demod88/1(Input Signal)
  Analog Filter Design221/1 -> SSB Demod60/1(Input Signal)
  Analog Filter Design234/1 -> Add6/8
  Analog Filter Design252/1 -> Add7/7
  Analog Filter Design235/1 -> SSB Demod67/1(Input Signal)
  Analog Filter Design132/1 -> SSB Demod15/1(Input Signal)
  Analog Filter Design120/1 -> SSB Demod9/1(Input Signal)
  Analog Filter Design131/1 -> Add1/6
  Analog Filter Design227/1 -> SSB Demod63/1(Input Signal)
  Analog Filter Design188/1 -> SSB Demod43/1(Input Signal)
  Analog Filter Design223/1 -> SSB Demod61/1(Input Signal)
  Analog Filter Design158/1 -> SSB Demod28/1(Input Signal)
  Analog Filter Design239/1 -> SSB Demod69/1(Input Signal)
  Analog Filter Design123/1 -> Add1/2
  Analog Filter Design217/1 -> SSB Demod58/1(Input Signal)
  Analog Filter Design265/1 -> SSB Demod82/1(Input Signal)
  Analog Filter Design299/1 -> SSB Demod99/1(Input Signal)
  Analog Filter Design124/1 -> SSB Demod11/1(Input Signal)
  Analog Filter Design135/1 -> Add1/8
  Analog Filter Design298/1 -> Add9/10
  Analog Filter Design111/1 -> Add/6
  Analog Filter Design230/1 -> Add6/6
  Analog Filter Design196/1 -> SSB Demod47/1(Input Signal)
  Analog Filter Design243/1 -> SSB Demod71/1(Input Signal)
  Analog Filter Design194/1 -> SSB Demod46/1(Input Signal)
  Analog Filter Design231/1 -> SSB Demod65/1(Input Signal)
  Analog Filter Design127/1 -> Add1/4
  Analog Filter Design168/1 -> SSB Demod33/1(Input Signal)
  Analog Filter Design191/1 -> Add4/6
  Analog Filter Design264/1 -> Add8/3
  Analog Filter Design237/1 -> SSB Demod68/1(Input Signal)
  Analog Filter Design245/1 -> SSB Demod72/1(Input Signal)
  Analog Filter Design257/1 -> SSB Demod78/1(Input Signal)
  Analog Filter Design291/1 -> SSB Demod95/1(Input Signal)
  Analog Filter Design139/1 -> Add1/10
  Analog Filter Design141/1 -> Add2/1
  Analog Filter Design159/1 -> Add2/10
  Analog Filter Design156/1 -> SSB Demod27/1(Input Signal)
  Analog Filter Design262/1 -> Add8/2
  Analog Filter Design278/1 -> Add8/10
  Analog Filter Design176/1 -> SSB Demod37/1(Input Signal)
  Analog Filter Design108/1 -> SSB Demod3/1(Input Signal)
  Analog Filter Design229/1 -> SSB Demod64/1(Input Signal)
  Analog Filter Design201/1 -> SSB Demod50/1(Input Signal)
  Analog Filter Design211/1 -> SSB Demod55/1(Input Signal)
  Analog Filter Design288/1 -> Add9/5
  Analog Filter Design295/1 -> SSB Demod97/1(Input Signal)
  Analog Filter Design104/1 -> SSB Demod1/1(Input Signal)
  Analog Filter Design269/1 -> SSB Demod84/1(Input Signal)
  Analog Filter Design112/1 -> SSB Demod5/1(Input Signal)
  Analog Filter Design192/1 -> SSB Demod45/1(Input Signal)
  Analog Filter Design261/1 -> SSB Demod80/1(Input Signal)
  Analog Filter Design134/1 -> SSB Demod16/1(Input Signal)
  Analog Filter Design143/1 -> Add2/2
  Analog Filter Design209/1 -> SSB Demod54/1(Input Signal)
  Analog Filter Design199/1 -> Add4/10
  Analog Filter Design285/1 -> SSB Demod92/1(Input Signal)
  Analog Filter Design164/1 -> SSB Demod31/1(Input Signal)
  Analog Filter Design259/1 -> SSB Demod79/1(Input Signal)
  Analog Filter Design241/1 -> SSB Demod70/1(Input Signal)
  Analog Filter Design275/1 -> SSB Demod87/1(Input Signal)
  Analog Filter Design205/1 -> SSB Demod52/1(Input Signal)
  Analog Filter Design294/1 -> Add9/8
  Analog Filter Design272/1 -> Add8/7
  Analog Filter Design161/1 -> Add3/1
  Analog Filter Design110/1 -> SSB Demod4/1(Input Signal)
  Analog Filter Design250/1 -> Add7/6
  Analog Filter Design200/1 -> SSB Demod49/1(Input Signal)
  SSB Modulator43/1(Out1) -> Analog Filter Design187/1
  Add2/1 -> Add10/3
  SSB Demod/1(Out1) -> Analog Filter Design1/1
  SSB Demod15/1(Out1) -> Analog Filter Design17/1
  message signal71/1 -> SSB Modulator71/1(Input Signal)
  SSB Demod54/1(Out1) -> Analog Filter Design95/1
  message signal93/1 -> SSB Modulator93/1(Input Signal)
  SSB Modulator48/1(Out1) -> Analog Filter Design197/1
  Analog Filter Design174/1 -> SSB Demod36/1(Input Signal)
  Analog Filter Design190/1 -> SSB Demod44/1(Input Signal)
  message signal83/1 -> SSB Modulator83/1(Input Signal)
  SSB Modulator77/1(Out1) -> Analog Filter Design254/1
  Analog Filter Design279/1 -> SSB Demod89/1(Input Signal)
  SSB Modulator59/1(Out1) -> Analog Filter Design218/1
  Analog Filter Design125/1 -> Add1/3
  SSB Modulator7/1(Out1) -> Analog Filter Design115/1
  message signal90/1 -> SSB Modulator90/1(Input Signal)
  SSB Modulator23/1(Out1) -> Analog Filter Design147/1
  message signal8/1 -> SSB Modulator8/1(Input Signal)
  SSB Modulator24/1(Out1) -> Analog Filter Design149/1
  message signal68/1 -> SSB Modulator68/1(Input Signal)
  SSB Demod35/1(Out1) -> Analog Filter Design37/1
  message signal15/1 -> SSB Modulator15/1(Input Signal)
  message signal66/1 -> SSB Modulator66/1(Input Signal)
  SSB Modulator98/1(Out1) -> Analog Filter Design296/1
  SSB Demod17/1(Out1) -> Analog Filter Design19/1
  Add3/1 -> Add10/4
  Analog Filter Design173/1 -> Add3/7
  Analog Filter Design121/1 -> Add1/1
  SSB Demod96/1(Out1) -> Analog Filter Design93/1
  message signal42/1 -> SSB Modulator42/1(Input Signal)
  message signal28/1 -> SSB Modulator28/1(Input Signal)
  message signal70/1 -> SSB Modulator70/1(Input Signal)
  Add9/1 -> Add10/10
  SSB Modulator69/1(Out1) -> Analog Filter Design238/1
  SSB Demod60/1(Out1) -> Analog Filter Design53/1
  message signal35/1 -> SSB Modulator35/1(Input Signal)
  SSB Modulator4/1(Out1) -> Analog Filter Design109/1
  SSB Demod70/1(Out1) -> Analog Filter Design64/1
  SSB Modulator56/1(Out1) -> Analog Filter Design212/1
  SSB Demod76/1(Out1) -> Analog Filter Design71/1
  SSB Demod28/1(Out1) -> Analog Filter Design30/1
  message signal77/1 -> SSB Modulator77/1(Input Signal)
  SSB Modulator19/1(Out1) -> Analog Filter Design139/1
  SSB Modulator66/1(Out1) -> Analog Filter Design232/1
  SSB Demod20/1(Out1) -> Analog Filter Design21/1
  SSB Modulator60/1(Out1) -> Analog Filter Design220/1
  Analog Filter Design281/1 -> SSB Demod90/1(Input Signal)
  SSB Demod3/1(Out1) -> Analog Filter Design4/1
  SSB Demod64/1(Out1) -> Analog Filter Design58/1
  Analog Filter Design296/1 -> Add9/9
  message signal86/1 -> SSB Modulator86/1(Input Signal)
  SSB Modulator41/1(Out1) -> Analog Filter Design183/1
  SSB Modulator64/1(Out1) -> Analog Filter Design228/1
  Analog Filter Design236/1 -> Add6/9
  SSB Demod36/1(Out1) -> Analog Filter Design38/1
  Analog Filter Design122/1 -> SSB Demod10/1(Input Signal)
  Analog Filter Design154/1 -> SSB Demod26/1(Input Signal)
  SSB Modulator32/1(Out1) -> Analog Filter Design165/1
  SSB Demod7/1(Out1) -> Analog Filter Design8/1
  Analog Filter Design256/1 -> Add7/9
  message signal97/1 -> SSB Modulator97/1(Input Signal)
  message signal51/1 -> SSB Modulator51/1(Input Signal)
  Analog Filter Design116/1 -> SSB Demod7/1(Input Signal)
  message signal45/1 -> SSB Modulator45/1(Input Signal)
  SSB Demod51/1(Out1) -> Analog Filter Design62/1
  SSB Modulator22/1(Out1) -> Analog Filter Design145/1
  Add/1 -> Add10/1
  SSB Modulator81/1(Out1) -> Analog Filter Design262/1
  SSB Demod53/1(Out1) -> Analog Filter Design84/1
  Analog Filter Design114/1 -> SSB Demod6/1(Input Signal)
  message signal18/1 -> SSB Modulator18/1(Input Signal)
  SSB Demod19/1(Out1) -> Analog Filter Design12/1
  SSB Demod11/1(Out1) -> Analog Filter Design13/1
  message signal40/1 -> SSB Modulator40/1(Input Signal)
  SSB Modulator83/1(Out1) -> Analog Filter Design266/1
  SSB Demod8/1(Out1) -> Analog Filter Design9/1
  Analog Filter Design214/1 -> Add5/8
  message signal94/1 -> SSB Modulator94/1(Input Signal)
  SSB Modulator26/1(Out1) -> Analog Filter Design153/1
  SSB Modulator40/1(Out1) -> Analog Filter Design181/1
  SSB Demod92/1(Out1) -> Analog Filter Design89/1
  message signal33/1 -> SSB Modulator33/1(Input Signal)
  SSB Demod49/1(Out1) -> Analog Filter Design42/1
  SSB Demod97/1(Out1) -> Analog Filter Design94/1
  SSB Demod1/1(Out1) -> Analog Filter Design2/1
  Analog Filter Design140/1 -> SSB Demod19/1(Input Signal)
  SSB Modulator3/1(Out1) -> Analog Filter Design107/1
  SSB Modulator20/1(Out1) -> Analog Filter Design141/1
  Analog Filter Design290/1 -> Add9/6
  message signal84/1 -> SSB Modulator84/1(Input Signal)
  message signal63/1 -> SSB Modulator63/1(Input Signal)
  SSB Demod22/1(Out1) -> Analog Filter Design24/1
  SSB Modulator1/1(Out1) -> BPF 2/1
  SSB Demod16/1(Out1) -> Analog Filter Design18/1
  SSB Modulator28/1(Out1) -> Analog Filter Design157/1
  SSB Demod89/1(Out1) -> Analog Filter Design76/1
  SSB Demod80/1(Out1) -> Analog Filter Design75/1
  Add4/1 -> Add10/5
  message signal98/1 -> SSB Modulator98/1(Input Signal)
  message signal29/1 -> SSB Modulator29/1(Input Signal)
  SSB Modulator35/1(Out1) -> Analog Filter Design171/1
  SSB Modulator73/1(Out1) -> Analog Filter Design246/1
  SSB Demod25/1(Out1) -> Analog Filter Design27/1
  SSB Demod55/1(Out1) -> Analog Filter Design97/1
  SSB Demod88/1(Out1) -> Analog Filter Design85/1
  SSB Modulator46/1(Out1) -> Analog Filter Design193/1
  SSB Demod71/1(Out1) -> Analog Filter Design66/1
  SSB Demod33/1(Out1) -> Analog Filter Design35/1
  SSB Demod12/1(Out1) -> Analog Filter Design14/1
  SSB Demod41/1(Out1) -> Analog Filter Design43/1
  message signal14/1 -> SSB Modulator14/1(Input Signal)
  SSB Modulator95/1(Out1) -> Analog Filter Design290/1
  SSB Modulator52/1(Out1) -> Analog Filter Design204/1
  SSB Modulator84/1(Out1) -> Analog Filter Design268/1
  SSB Demod72/1(Out1) -> Analog Filter Design67/1
  SSB Modulator85/1(Out1) -> Analog Filter Design270/1
  SSB Modulator25/1(Out1) -> Analog Filter Design151/1
  message signal5/1 -> SSB Modulator5/1(Input Signal)
  Analog Filter Design228/1 -> Add6/5
  message signal59/1 -> SSB Modulator59/1(Input Signal)
  SSB Modulator99/1(Out1) -> Analog Filter Design298/1
  Analog Filter Design271/1 -> SSB Demod85/1(Input Signal)
  message signal2/1 -> SSB Modulator2/1(Input Signal)
  SSB Demod46/1(Out1) -> Analog Filter Design48/1
  SSB Modulator74/1(Out1) -> Analog Filter Design248/1
  SSB Demod40/1(Out1) -> Analog Filter Design41/1
  message signal57/1 -> SSB Modulator57/1(Input Signal)
  message signal4/1 -> SSB Modulator4/1(Input Signal)
  SSB Demod95/1(Out1) -> Analog Filter Design92/1
  SSB Modulator27/1(Out1) -> Analog Filter Design155/1
  SSB Demod6/1(Out1) -> Analog Filter Design7/1
  message signal12/1 -> SSB Modulator12/1(Input Signal)
  SSB Demod77/1(Out1) -> Analog Filter Design72/1
  message signal41/1 -> SSB Modulator41/1(Input Signal)
  SSB Demod78/1(Out1) -> Analog Filter Design74/1
  SSB Demod48/1(Out1) -> Analog Filter Design50/1
  SSB Demod27/1(Out1) -> Analog Filter Design29/1
  SSB Modulator93/1(Out1) -> Analog Filter Design286/1
  Analog Filter Design270/1 -> Add8/6
  SSB Demod21/1(Out1) -> Analog Filter Design23/1
  Analog Filter Design136/1 -> SSB Demod17/1(Input Signal)
  SSB Demod87/1(Out1) -> Analog Filter Design83/1
  message signal47/1 -> SSB Modulator47/1(Input Signal)
  message signal21/1 -> SSB Modulator21/1(Input Signal)
  SSB Demod2/1(Out1) -> Analog Filter Design3/1
  message signal6/1 -> SSB Modulator6/1(Input Signal)
  message signal60/1 -> SSB Modulator60/1(Input Signal)
  Analog Filter Design292/1 -> Add9/7
  SSB Modulator61/1(Out1) -> Analog Filter Design222/1
  SSB Modulator70/1(Out1) -> Analog Filter Design240/1
  SSB Demod23/1(Out1) -> Analog Filter Design25/1
  Add5/1 -> Add10/6
  SSB Modulator71/1(Out1) -> Analog Filter Design242/1
  Add1/1 -> Add10/2
  SSB Modulator8/1(Out1) -> Analog Filter Design117/1
  Analog Filter Design/1 -> Add5/1
  Analog Filter Design212/1 -> Add5/7
  SSB Demod29/1(Out1) -> Analog Filter Design22/1
  Analog Filter Design242/1 -> Add7/2
  message signal27/1 -> SSB Modulator27/1(Input Signal)
  message signal17/1 -> SSB Modulator17/1(Input Signal)
  message signal37/1 -> SSB Modulator37/1(Input Signal)
  SSB Modulator18/1(Out1) -> Analog Filter Design137/1
  Analog Filter Design218/1 -> Add5/10
  SSB Demod94/1(Out1) -> Analog Filter Design91/1
  Analog Filter Design119/1 -> Add/10
  SSB Modulator29/1(Out1) -> Analog Filter Design159/1
  Add6/1 -> Add10/7
  Analog Filter Design169/1 -> Add3/5
  message signal36/1 -> SSB Modulator36/1(Input Signal)
  SSB Demod39/1(Out1) -> Analog Filter Design32/1
  SSB Modulator86/1(Out1) -> Analog Filter Design272/1
  Analog Filter Design197/1 -> Add4/9
  SSB Modulator31/1(Out1) -> Analog Filter Design163/1
  message signal75/1 -> SSB Modulator75/1(Input Signal)
  SSB Modulator50/1(Out1) -> Analog Filter Design/1
  message signal9/1 -> SSB Modulator9/1(Input Signal)
  Analog Filter Design283/1 -> SSB Demod91/1(Input Signal)
  Analog Filter Design222/1 -> Add6/2
  SSB Modulator63/1(Out1) -> Analog Filter Design226/1
  Analog Filter Design276/1 -> Add8/9
  message signal79/1 -> SSB Modulator79/1(Input Signal)
  SSB Modulator62/1(Out1) -> Analog Filter Design224/1
  Analog Filter Design105/1 -> Add/3
  SSB Demod83/1(Out1) -> Analog Filter Design79/1
  message signal43/1 -> SSB Modulator43/1(Input Signal)
  SSB Demod90/1(Out1) -> Analog Filter Design86/1
  Analog Filter Design282/1 -> Add9/2
  message signal76/1 -> SSB Modulator76/1(Input Signal)
  SSB Modulator11/1(Out1) -> Analog Filter Design123/1
  Analog Filter Design137/1 -> Add1/9
  Analog Filter Design149/1 -> Add2/5
  Analog Filter Design165/1 -> Add3/3
  Analog Filter Design204/1 -> Add5/3
  Analog Filter Design267/1 -> SSB Demod83/1(Input Signal)
  SSB Modulator/1(Out1) -> BPF1/1
  Analog Filter Design233/1 -> SSB Demod66/1(Input Signal)
  message signal34/1 -> SSB Modulator34/1(Input Signal)
  Analog Filter Design297/1 -> SSB Demod98/1(Input Signal)
  Analog Filter Design240/1 -> Add7/1
  Analog Filter Design163/1 -> Add3/2
  Analog Filter Design247/1 -> SSB Demod73/1(Input Signal)
  SSB Demod75/1(Out1) -> Analog Filter Design70/1
  Analog Filter Design244/1 -> Add7/3
  Analog Filter Design177/1 -> Add3/9
  message signal96/1 -> SSB Modulator96/1(Input Signal)
  SSB Demod47/1(Out1) -> Analog Filter Design49/1
  message signal87/1 -> SSB Modulator87/1(Input Signal)
  Analog Filter Design117/1 -> Add/9
  Analog Filter Design293/1 -> SSB Demod96/1(Input Signal)
  Analog Filter Design179/1 -> Add3/10
  Add7/1 -> Add10/8
  SSB Demod93/1(Out1) -> Analog Filter Design90/1
  SSB Modulator5/1(Out1) -> Analog Filter Design111/1
  Analog Filter Design151/1 -> Add2/6
  SSB Demod32/1(Out1) -> Analog Filter Design34/1
  message signal16/1 -> SSB Modulator16/1(Input Signal)
  Analog Filter Design118/1 -> SSB Demod8/1(Input Signal)
  SSB Modulator57/1(Out1) -> Analog Filter Design214/1
  Analog Filter Design215/1 -> SSB Demod57/1(Input Signal)
  SSB Demod74/1(Out1) -> Analog Filter Design69/1
  message signal54/1 -> SSB Modulator54/1(Input Signal)
  Analog Filter Design246/1 -> Add7/4
  SSB Demod81/1(Out1) -> Analog Filter Design77/1
  Analog Filter Design160/1 -> SSB Demod29/1(Input Signal)
  SSB Modulator80/1(Out1) -> Analog Filter Design260/1
  SSB Modulator47/1(Out1) -> Analog Filter Design195/1
  message signal32/1 -> SSB Modulator32/1(Input Signal)
  Analog Filter Design208/1 -> Add5/5
  SSB Demod85/1(Out1) -> Analog Filter Design81/1
  Analog Filter Design166/1 -> SSB Demod32/1(Input Signal)
  SSB Modulator68/1(Out1) -> Analog Filter Design236/1
  Analog Filter Design175/1 -> Add3/8
  SSB Demod45/1(Out1) -> Analog Filter Design47/1
  AWGN Channel/1 -> Analog Filter Design201/1, Analog Filter Design200/1, Analog Filter Design196/1, Analog Filter Design194/1, Analog Filter Design192/1, Analog Filter Design190/1, Analog Filter Design188/1, Analog Filter Design186/1, Analog Filter Design184/1, Analog Filter Design178/1, Analog Filter Design176/1, Analog Filter Design174/1, Analog Filter Design166/1, Analog Filter Design164/1, Analog Filter Design162/1, Analog Filter Design160/1, Analog Filter Design156/1, Analog Filter Design154/1, Analog Filter Design152/1, Analog Filter Design150/1, Analog Filter Design148/1, Analog Filter Design146/1, Analog Filter Design144/1, Analog Filter Design142/1, Analog Filter Design138/1, Analog Filter Design134/1, Analog Filter Design132/1, Analog Filter Design128/1, Analog Filter Design126/1, Analog Filter Design124/1, Analog Filter Design122/1, Analog Filter Design118/1, Analog Filter Design116/1, Analog Filter Design114/1, Analog Filter Design112/1, Analog Filter Design110/1, Analog Filter Design108/1, Analog Filter Design106/1, Analog Filter Design102/1, Analog Filter Design104/1, Analog Filter Design120/1, Analog Filter Design130/1, Analog Filter Design136/1, Analog Filter Design140/1, Analog Filter Design158/1, Analog Filter Design168/1, Analog Filter Design170/1, Analog Filter Design172/1, Analog Filter Design180/1, Analog Filter Design182/1, Analog Filter Design198/1, Analog Filter Design203/1, Analog Filter Design207/1, Analog Filter Design209/1, Analog Filter Design211/1, Analog Filter Design215/1, Analog Filter Design217/1, Analog Filter Design219/1, Analog Filter Design221/1, Analog Filter Design223/1, Analog Filter Design225/1, Analog Filter Design231/1, Analog Filter Design233/1, Analog Filter Design235/1, Analog Filter Design237/1, Analog Filter Design239/1, Analog Filter Design241/1, Analog Filter Design243/1, Analog Filter Design245/1, Analog Filter Design247/1, Analog Filter Design249/1, Analog Filter Design251/1, Analog Filter Design253/1, Analog Filter Design255/1, Analog Filter Design257/1, Analog Filter Design259/1, Analog Filter Design261/1, Analog Filter Design263/1, Analog Filter Design265/1, Analog Filter Design267/1, Analog Filter Design269/1, Analog Filter Design271/1, Analog Filter Design273/1, Analog Filter Design275/1, Analog Filter Design277/1, Analog Filter Design279/1, Analog Filter Design283/1, Analog Filter Design285/1, Analog Filter Design287/1, Analog Filter Design289/1, Analog Filter Design291/1, Analog Filter Design293/1, Analog Filter Design295/1, Analog Filter Design299/1, Analog Filter Design297/1, Analog Filter Design281/1, Analog Filter Design229/1, Analog Filter Design227/1, Analog Filter Design213/1, Analog Filter Design205/1
  message signal82/1 -> SSB Modulator82/1(Input Signal)
  Analog Filter Design129/1 -> Add1/5
  Analog Filter Design268/1 -> Add8/5
  SSB Modulator78/1(Out1) -> Analog Filter Design256/1
  SSB Demod79/1(Out1) -> Analog Filter Design65/1
  message signal26/1 -> SSB Modulator26/1(Input Signal)
  message signal50/1 -> Scope1/1, SSB Modulator50/1(Input Signal)
  Analog Filter Design128/1 -> SSB Demod13/1(Input Signal)
  Analog Filter Design162/1 -> SSB Demod30/1(Input Signal)
  Add8/1 -> Add10/9
  message signal80/1 -> SSB Modulator80/1(Input Signal)
  SSB Demod56/1(Out1) -> Analog Filter Design98/1
  SSB Modulator44/1(Out1) -> Analog Filter Design189/1
  SSB Demod24/1(Out1) -> Analog Filter Design26/1
  message signal44/1 -> SSB Modulator44/1(Input Signal)
  Analog Filter Design144/1 -> SSB Demod21/1(Input Signal)
  SSB Demod84/1(Out1) -> Analog Filter Design80/1
  SSB Modulator97/1(Out1) -> Analog Filter Design294/1
  Analog Filter Design106/1 -> SSB Demod2/1(Input Signal)
  SSB Modulator12/1(Out1) -> Analog Filter Design125/1
  SSB Demod66/1(Out1) -> Analog Filter Design60/1
  SSB Demod86/1(Out1) -> Analog Filter Design82/1
  Analog Filter Design152/1 -> SSB Demod25/1(Input Signal)
  SSB Demod18/1(Out1) -> Analog Filter Design20/1
  message signal64/1 -> SSB Modulator64/1(Input Signal)
  SSB Modulator33/1(Out1) -> Analog Filter Design167/1
  SSB Modulator39/1(Out1) -> Analog Filter Design179/1
  SSB Modulator91/1(Out1) -> Analog Filter Design282/1
  SSB Demod69/1(Out1) -> Analog Filter Design54/1
  Analog Filter Design102/1 -> SSB Demod/1(Input Signal)
  SSB Modulator2/1(Out1) -> Analog Filter Design105/1
  SSB Demod44/1(Out1) -> Analog Filter Design46/1
  message signal31/1 -> SSB Modulator31/1(Input Signal)
  SSB Modulator65/1(Out1) -> Analog Filter Design230/1
  SSB Demod9/1(Out1) -> Analog Filter Design10/1
  SSB Demod50/1(Out1) -> Analog Filter Design51/1
  message signal88/1 -> SSB Modulator88/1(Input Signal)
  message signal23/1 -> SSB Modulator23/1(Input Signal)
  message signal69/1 -> SSB Modulator69/1(Input Signal)
  Analog Filter Design186/1 -> SSB Demod42/1(Input Signal)
  message signal92/1 -> SSB Modulator92/1(Input Signal)
  SSB Modulator15/1(Out1) -> Analog Filter Design131/1
  SSB Demod98/1(Out1) -> Analog Filter Design96/1
  SSB Demod26/1(Out1) -> Analog Filter Design28/1
  SSB Modulator82/1(Out1) -> Analog Filter Design264/1
  message signal7/1 -> SSB Modulator7/1(Input Signal)
  message signal30/1 -> SSB Modulator30/1(Input Signal)
  SSB Modulator94/1(Out1) -> Analog Filter Design288/1
  SSB Demod59/1(Out1) -> Analog Filter Design52/1
  SSB Demod14/1(Out1) -> Analog Filter Design16/1
  SSB Modulator76/1(Out1) -> Analog Filter Design252/1
  SSB Demod73/1(Out1) -> Analog Filter Design68/1
  message signal11/1 -> SSB Modulator11/1(Input Signal)
  message signal73/1 -> SSB Modulator73/1(Input Signal)
  SSB Modulator96/1(Out1) -> Analog Filter Design292/1
  message signal52/1 -> SSB Modulator52/1(Input Signal)
  Analog Filter Design263/1 -> SSB Demod81/1(Input Signal)
  Analog Filter Design178/1 -> SSB Demod38/1(Input Signal)
  message signal24/1 -> SSB Modulator24/1(Input Signal)
  SSB Modulator10/1(Out1) -> Analog Filter Design121/1
  message signal38/1 -> SSB Modulator38/1(Input Signal)
  Analog Filter Design150/1 -> SSB Demod24/1(Input Signal)
  SSB Demod37/1(Out1) -> Analog Filter Design39/1
  SSB Modulator51/1(Out1) -> Analog Filter Design202/1
  SSB Modulator58/1(Out1) -> Analog Filter Design216/1
  message signal25/1 -> SSB Modulator25/1(Input Signal)
  SSB Demod5/1(Out1) -> Analog Filter Design6/1
  message signal74/1 -> SSB Modulator74/1(Input Signal)
  SSB Modulator9/1(Out1) -> Analog Filter Design119/1
  message signal58/1 -> SSB Modulator58/1(Input Signal)
  message signal67/1 -> SSB Modulator67/1(Input Signal)
  SSB Demod30/1(Out1) -> Analog Filter Design31/1
  Analog Filter Design273/1 -> SSB Demod86/1(Input Signal)
  SSB Modulator34/1(Out1) -> Analog Filter Design169/1
  SSB Modulator45/1(Out1) -> Analog Filter Design191/1
  SSB Modulator89/1(Out1) -> Analog Filter Design278/1
  SSB Modulator17/1(Out1) -> Analog Filter Design135/1
  SSB Demod43/1(Out1) -> Analog Filter Design45/1
  SSB Demod57/1(Out1) -> Analog Filter Design99/1
  SSB Demod62/1(Out1) -> Analog Filter Design56/1
  Analog Filter Design254/1 -> Add7/8
  message signal1/1 -> SSB Modulator1/1(Input Signal)
  message signal78/1 -> SSB Modulator78/1(Input Signal)
  SSB Demod91/1(Out1) -> Analog Filter Design88/1
  SSB Modulator36/1(Out1) -> Analog Filter Design173/1
  SSB Modulator92/1(Out1) -> Analog Filter Design284/1
  message signal20/1 -> SSB Modulator20/1(Input Signal)
  message signal95/1 -> SSB Modulator95/1(Input Signal)
  Analog Filter Design126/1 -> SSB Demod12/1(Input Signal)
  SSB Demod63/1(Out1) -> Analog Filter Design57/1
  message signal19/1 -> SSB Modulator19/1(Input Signal)
  SSB Demod82/1(Out1) -> Analog Filter Design78/1
  SSB Modulator67/1(Out1) -> Analog Filter Design234/1
  SSB Demod31/1(Out1) -> Analog Filter Design33/1
  message signal62/1 -> SSB Modulator62/1(Input Signal)
  message signal61/1 -> SSB Modulator61/1(Input Signal)
  SSB Modulator75/1(Out1) -> Analog Filter Design250/1
  Analog Filter Design225/1 -> SSB Demod62/1(Input Signal)
  BPF 2/1 -> Add/2
  SSB Demod10/1(Out1) -> Analog Filter Design11/1
  message signal46/1 -> SSB Modulator46/1(Input Signal)
  SSB Modulator54/1(Out1) -> Analog Filter Design208/1
  SSB Demod52/1(Out1) -> Analog Filter Design73/1
  Analog Filter Design184/1 -> SSB Demod41/1(Input Signal)
  SSB Modulator87/1(Out1) -> Analog Filter Design274/1
  SSB Modulator37/1(Out1) -> Analog Filter Design175/1
  Analog Filter Design193/1 -> Add4/7
  message signal10/1 -> SSB Modulator10/1(Input Signal)
  SSB Demod13/1(Out1) -> Analog Filter Design15/1
  SSB Demod61/1(Out1) -> Analog Filter Design55/1
  SSB Modulator88/1(Out1) -> Analog Filter Design276/1
  message signal56/1 -> SSB Modulator56/1(Input Signal)
  message signal85/1 -> SSB Modulator85/1(Input Signal)
  SSB Modulator16/1(Out1) -> Analog Filter Design133/1
  Analog Filter Design226/1 -> Add6/4
  SSB Demod38/1(Out1) -> Analog Filter Design40/1
  SSB Demod58/1(Out1) -> Analog Filter Design100/1
  SSB Demod42/1(Out1) -> Analog Filter Design44/1
  Analog Filter Design187/1 -> Add4/4
  SSB Modulator42/1(Out1) -> Analog Filter Design185/1
  message signal53/1 -> SSB Modulator53/1(Input Signal)
  SSB Demod67/1(Out1) -> Analog Filter Design61/1
  Analog Filter Design198/1 -> SSB Demod48/1(Input Signal)
  message signal3/1 -> SSB Modulator3/1(Input Signal)
  message signal48/1 -> SSB Modulator48/1(Input Signal)
  message signal65/1 -> SSB Modulator65/1(Input Signal)
  SSB Demod99/1(Out1) -> Analog Filter Design87/1
  message signal39/1 -> SSB Modulator39/1(Input Signal)
  SSB Modulator38/1(Out1) -> Analog Filter Design177/1
  SSB Modulator14/1(Out1) -> Analog Filter Design129/1
  message signal91/1 -> SSB Modulator91/1(Input Signal)
  message signal55/1 -> SSB Modulator55/1(Input Signal)
  SSB Modulator6/1(Out1) -> Analog Filter Design113/1
  SSB Modulator90/1(Out1) -> Analog Filter Design280/1
  message signal72/1 -> SSB Modulator72/1(Input Signal)
  Analog Filter Design167/1 -> Add3/4
  message signal49/1 -> SSB Modulator49/1(Input Signal)
  SSB Modulator13/1(Out1) -> Analog Filter Design127/1
  SSB Modulator79/1(Out1) -> Analog Filter Design258/1
  SSB Modulator72/1(Out1) -> Analog Filter Design244/1
  SSB Modulator49/1(Out1) -> Analog Filter Design199/1
  Analog Filter Design253/1 -> SSB Demod76/1(Input Signal)
  SSB Modulator53/1(Out1) -> Analog Filter Design206/1
  message signal89/1 -> SSB Modulator89/1(Input Signal)
  SSB Demod65/1(Out1) -> Analog Filter Design59/1
  SSB Demod68/1(Out1) -> Analog Filter Design63/1
  message signal22/1 -> SSB Modulator22/1(Input Signal)
  SSB Demod4/1(Out1) -> Analog Filter Design5/1
  Analog Filter Design274/1 -> Add8/8
  SSB Demod34/1(Out1) -> Analog Filter Design36/1
  message signal13/1 -> SSB Modulator13/1(Input Signal)
  Analog Filter Design258/1 -> Add7/10
  BPF1/1 -> Add/1
  Analog Filter Design249/1 -> SSB Demod74/1(Input Signal)
  message signal/1 -> Scope/1, SSB Modulator/1(Input Signal)
  SSB Modulator30/1(Out1) -> Analog Filter Design161/1
  message signal81/1 -> SSB Modulator81/1(Input Signal)
  Analog Filter Design87/1 -> Scope2/2
  message signal99/1 -> Scope2/1, SSB Modulator99/1(Input Signal)
  SSB Modulator21/1(Out1) -> Analog Filter Design143/1
  SSB Modulator55/1(Out1) -> Analog Filter Design210/1
  Add10/1 -> AWGN Channel/1
